simulink model "Lin_Model_Control"  (R2018a)
settings: Solver=VariableStepAuto  StartTime=0.0  StopTime=40  RelTol=1e-3
values from neighbouring files (symbols this model uses):
  A = zeros(15,15)    [Quadrotor_Model.m]
  A_ad = [zeros(3,3), eye(3) ... (first row only)    [Admittance.m]
  B = zeros(15,7)    [Quadrotor_Model.m]
  B_ad = [zeros(3,3), zeros(3,3) ... (first row only)    [Admittance.m]
  C = zeros(6,15)    [Quadrotor_Model.m]
  C_ad = [eye(3), zeros(3,3)]    [Admittance.m]
  D = zeros(6,7)    [Quadrotor_Model.m]
  D_ad = zeros(3,6)    [Admittance.m]
  init_state = [x0 y0 z0  vx0 vy0 vz0 phi0 theta0 psi0 p0 q0 r0 tau_phi0 tau_theta0 tau_psi0]'    [Quadrotor_Model.m]
  p = menu('Choose the problem: 1 for trajectory tracking and 2 for regulation', 1,2)    [Admittance.m]
  par = [m;m1;Ix;Iy;Iz;Ir;Om_r;d;l;g]    [Quadrotor_Model.m]
undefined symbols (not defined in the file or in its folder): Ak, Bk, Ck, Continuous, Dk, Time, Tn, V, v
libraries: ctrlSharedLib x1
settings Model: Creator=Pimentel  LastModifiedBy=Pimentel

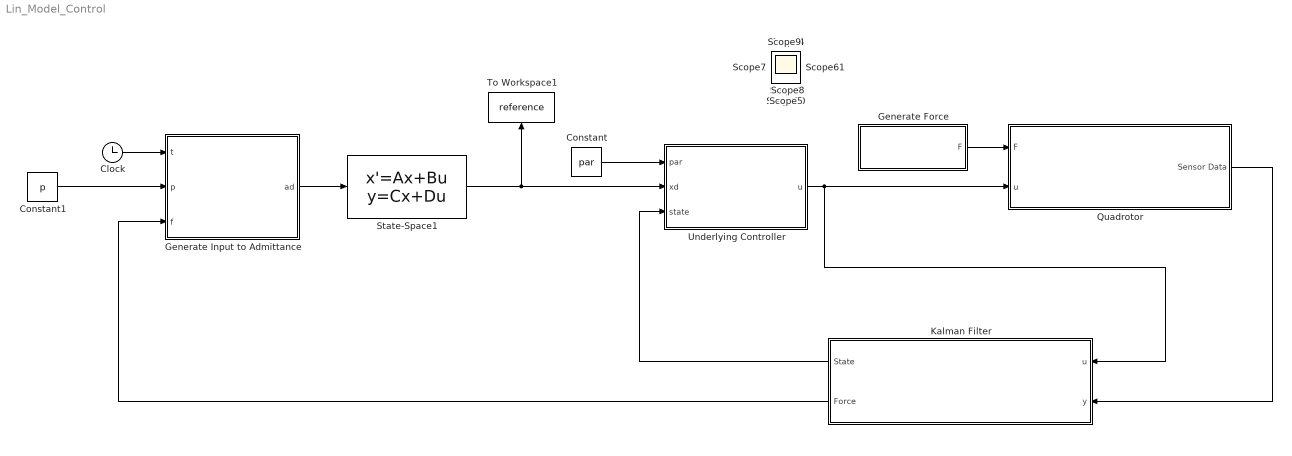
== system Lin_Model_Control ==
  Clock : Clock
  Constant : Constant  Value=par
  Constant1 : Constant  Value=p
  Generate Force : Subsystem
  "Generate Input to Admittance " : MATLAB Function  TreatAsAtomicUnit=on
  Kalman Filter : Subsystem
  "Quadrotor " : Subsystem
  State-Space1 : StateSpace  A=A_ad  B=B_ad  C=C_ad  D=D_ad  InitialCondition=[0 0 0 0 0 0]
  To Workspace1 : ToWorkspace  VariableName=reference  SaveFormat=Structure With Time  SampleTime=-1
  Underlying Controller : MATLAB Function  TreatAsAtomicUnit=on
  Scope{,1..11} (12 alike) : Scope
  wires:
  Underlying Controller/1(u) -> "Quadrotor "/2("u "), Kalman Filter/1(u)
  Clock/1 -> "Generate Input to Admittance "/1(t)
  Constant/1 -> Underlying Controller/1(par)
  State-Space1/1 -> Underlying Controller/2(xd), To Workspace1/1
  "Generate Input to Admittance "/1(ad) -> State-Space1/1
  Kalman Filter/2(Force) -> "Generate Input to Admittance "/3(f)
  Kalman Filter/1(State) -> Underlying Controller/3(state)
  "Quadrotor "/1(Sensor Data) -> Kalman Filter/2(y)
  Generate Force/1(F) -> "Quadrotor "/1(F)
  Constant1/1 -> "Generate Input to Admittance "/2(p)

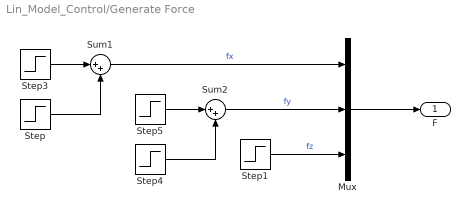
== system Lin_Model_Control/Generate Force ==
  Mux : Mux  Inputs=3
  Step : Step  Time=6  After=-3  SampleTime=0
  Step1 : Step  After=0  SampleTime=0
  Step3 : Step  After=3  SampleTime=0
  Step4 : Step  Time=6  After=-1  SampleTime=0
  Step5 : Step  SampleTime=0
  Sum1 : Sum  Inputs=|++
  Sum2 : Sum  Inputs=|++
  F : Outport
  wires:
  Mux/1 -> F/1
  Sum1/1 -> Mux/1  "fx"
  Step/1 -> Sum1/2
  Step1/1 -> Mux/3  "fz"
  Step3/1 -> Sum1/1
  Step4/1 -> Sum2/2
  Step5/1 -> Sum2/1
  Sum2/1 -> Mux/2  "fy"

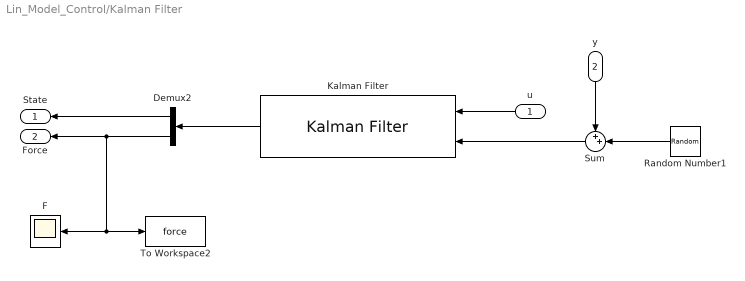
== system Lin_Model_Control/Kalman Filter ==
  u : Inport
  y : Inport  Port=2
  Demux2 : Demux  Outputs=[15, 3]
  F : Scope
  Kalman Filter : ctrlSharedLib/Kalman Filter  TimeDomain=Continuous-Time  UseCurrentEstimator=on  ModelSource=Individual A, B, C, D matrices  ModelSourceVariable=ss(0.95,1,1,0,1)  A=Ak  B=Bk  C=Ck  D=Dk  NumberOfStates=1  NumberOfInputs=1  NumberOfOutputs=1  InitialEstimateSource=Dialog  X0=0  P0=10  UseK=off  UseGH=off  NumberOfProcessNoiseInputs=1  G=1  TimeInvariantG=on  H=0  TimeInvariantH=on  Q=W  TimeInvariantQ=on  R=V  TimeInvariantR=on  N=0  TimeInvariantN=on  AddInputPort=on  AddEnablePort=off  OutputEstimatedY=off  OutputP=off  Ts=-1
      settings: SourceProductBaseCode=CT
  Random Number1 : RandomNumber  Mean=[0 0 0 0 0 0]  Variance=v  SampleTime=Tn
  Sum : Sum  Inputs=++|
  To Workspace2 : ToWorkspace  VariableName=force  SaveFormat=Structure With Time  SampleTime=-1
  State : Outport
  Force : Outport  Port=2
  wires:
  y/1 -> Sum/1
  Demux2/2 -> To Workspace2/1, F/1, Force/1
  Kalman Filter/1 -> Demux2/1
  Demux2/1 -> State/1
  Random Number1/1 -> Sum/2
  Sum/1 -> Kalman Filter/2
  u/1 -> Kalman Filter/1

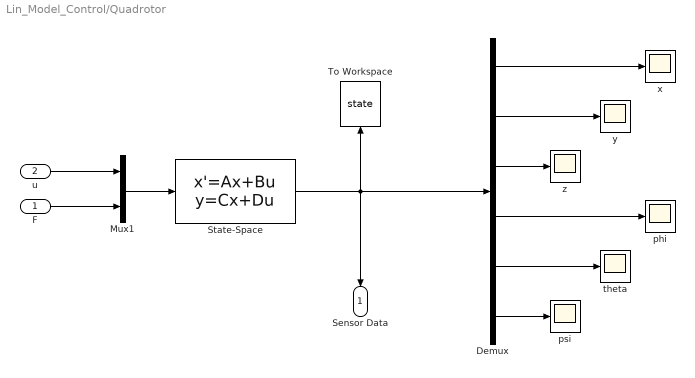
== system Lin_Model_Control/Quadrotor  ==
  F : Inport
  "u " : Inport  Port=2
  Demux : Demux  Outputs=6
  Mux1 : Mux  Inputs=2
  State-Space : StateSpace  A=A  B=B  C=C  D=D  InitialCondition=init_state
  To Workspace : ToWorkspace  VariableName=state  SaveFormat=Structure With Time  SampleTime=-1
  phi : Scope
  psi : Scope
  theta : Scope
  "x " : Scope
  y : Scope
  z : Scope
  Sensor Data : Outport
  wires:
  Demux/5 -> theta/1
  Demux/1 -> "x "/1
  Demux/4 -> phi/1
  F/1 -> Mux1/2
  Demux/6 -> psi/1
  "u "/1 -> Mux1/1
  State-Space/1 -> Demux/1, To Workspace/1, Sensor Data/1
  Mux1/1 -> State-Space/1
  Demux/3 -> z/1
  Demux/2 -> y/1

== matlab function Lin_Model_Control/Generate Input to Admittance  ==
  data: t input; p input; f input; ad output
function ad = generate(t,p,f)

if p == 1
    x_d = cos(t);
    y_d = sin(t);
    z_d = 0;
else
    x_d = 0;
    y_d = 0;
    z_d = 0;
end 

if f(1)>0.3
    fx = f(1);
else 
    fx = 0;
end

if f(2)>0.3
    fy = f(2);
else 
    fy = 0;
end

if f(3)>0.3
    fz = f(3);
else 
    fz = 0;    
end

ad = [x_d, y_d, z_d, fx, fy, fz]';

== matlab function Lin_Model_Control/Underlying Controller ==
  data: par input; xd input; state input; u output
function u = Pos_Att_Control(par, xd, state)

% Model Parameters 

m = par(1);
m1 = par(2);
Ix = par(3);
Iy = par(4);
Iz = par(5);
Ir = par(6);
Om_r = par(7);
d = par(8);
l = par(9);
g = par(10);

% State

x = state(1);
y = state(2);
z = state(3);
vx = state(4);
vy = state(5);
vz = state(6);
phi = state(7);
theta = state(8);
psi = state(9);
phi_dot = state(10);
theta_dot = state(11);
psi_dot = state(12);
tau_phi = state(13);
tau_theta = state(14);
tau_psi = state(15);

% Controller Gains 

kx_p = 20;
kx_d = 10;

ky_p = 20;
ky_d = 10;

kz_p = 20;
kz_d = 10;

k_phi = 20;
k_theta = 20;
k_psi = 1;

% Reference Trajectory
 
x_d = xd(1);
y_d = xd(2);
z_d = xd(3);

vx_d = 0;
vy_d = 0;
vz_d = 0;

% Altitude Control

T_Tilde = m*(g-kz_p*(z_d - z) - kz_d*(vz_d - vz));
T = T_Tilde/m - g;

% Attitude Control

theta_d = -1/g*(kx_p*(x_d - x) + kx_d*(vx_d - vx));
phi_d = 1/g*(ky_p*(y_d - y) + ky_d*(vy_d - vy));
psi_d = 0;

phi_dot_cmd = k_phi*(phi_d - phi);
theta_dot_cmd = k_theta*(theta_d - theta);
psi_dot_cmd = k_psi*(psi_d - psi);

u = [T, phi_dot_cmd, theta_dot_cmd, psi_dot_cmd]';
